simulink model "gravity"  (R2023a)
settings: Solver=FixedStepAuto  StartTime=0.0  StopTime=10.0  FixedStep=0.001  RelTol=1e-3
libraries: matrix_library x2
settings Model: Creator=romanos  LastModifiedBy=romanos
settings DataIOCC: ExternalInput="X_ecef,  R"  LoadExternalInput=on

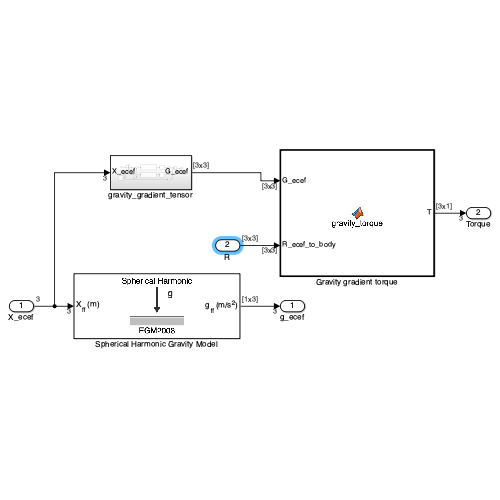
[thumbnail: Simulink's stored preview of the top-level diagram]
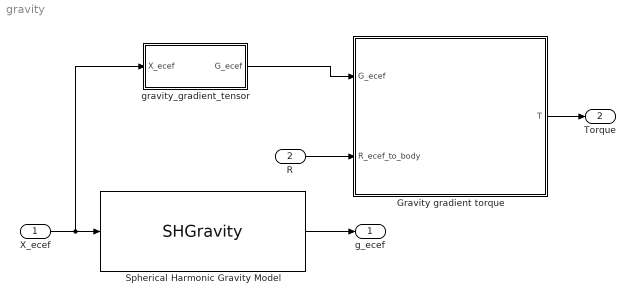
== system gravity ==
  X_ecef : Inport  PortDimensions=3
  R : Inport  Port=2  PortDimensions=[3 3]  Interpolate=off
  Gravity gradient torque : MATLAB Function  TreatAsAtomicUnit=on
  Spherical Harmonic Gravity Model : SHGravity
  gravity_gradient_tensor : Subsystem
  g_ecef : Outport  PortDimensions=3
  Torque : Outport  Port=2  PortDimensions=3
  wires:
  Gravity gradient torque/1(T) -> Torque/1
  X_ecef/1 -> Spherical Harmonic Gravity Model/1, gravity_gradient_tensor/1(X_ecef)
  Spherical Harmonic Gravity Model/1 -> g_ecef/1
  R/1 -> Gravity gradient torque/2(R_ecef_to_body)
  gravity_gradient_tensor/1(G_ecef) -> Gravity gradient torque/1(G_ecef)

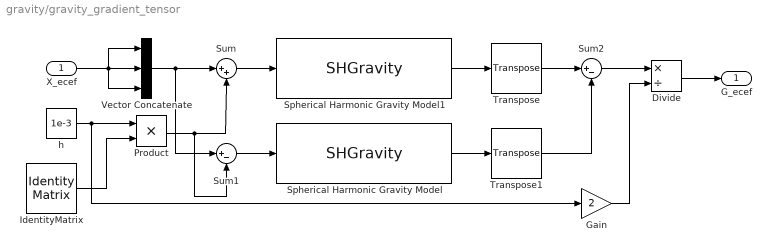
== system gravity/gravity_gradient_tensor ==
  X_ecef : Inport
  Divide : Product  Inputs=*/
  Gain : Gain  Gain=2
  IdentityMatrix : IdentityMatrix  OutputDimensions=3
  Product : Product
  Spherical Harmonic Gravity Model : SHGravity
  Spherical Harmonic Gravity Model1 : SHGravity
  Sum : Sum  Inputs=|++
  Sum1 : Sum  Inputs=|+-
  Sum2 : Sum  Inputs=|+-
  Transpose : matrix_library/Transpose
  Transpose1 : matrix_library/Transpose
  Vector Concatenate : Concatenate  NumInputs=3  Mode=Multidimensional array  ConcatenateDimension=2
  h : Constant  Value=1e-3
  G_ecef : Outport  PortDimensions=[3 3]
  wires:
  Divide/1 -> G_ecef/1
  Sum2/1 -> Divide/1
  Transpose/1 -> Sum2/1
  Gain/1 -> Divide/2
  Transpose1/1 -> Sum2/2
  Sum1/1 -> Spherical Harmonic Gravity Model/1
  Spherical Harmonic Gravity Model/1 -> Transpose1/1
  Sum/1 -> Spherical Harmonic Gravity Model1/1
  Product/1 -> Sum/2, Sum1/2
  h/1 -> Product/1, Gain/1
  Vector Concatenate/1 -> Sum1/1, Sum/1
  Spherical Harmonic Gravity Model1/1 -> Transpose/1
  IdentityMatrix/1 -> Product/2
  X_ecef/1 -> Vector Concatenate/1, Vector Concatenate/3, Vector Concatenate/2

== matlab function gravity/Gravity gradient torque ==
  data: G_ecef input; T output; R_ecef_to_body input; I parameter
function T   = gravity_torque(G_ecef, R_ecef_to_body, I) %#codegen
    G_body = R_ecef_to_body' * G_ecef * R_ecef_to_body;
    T = zeros(3,1);
    T(1) = G_body(2,3) * (I(3,3) - I(2,2)) + G_body(1,3) * I(1,2) - G_body(1,2) * I(1,3) + I(2,3) * (G_body(3,3) - G_body(2,2));
    T(2) = G_body(1,3) * (I(1,1) - I(3,3)) - G_body(2,3) * I(1,2) + G_body(1,2) * I(2,3) + I(1,3) * (G_body(1,1) - G_body(3,3));
    T(3) = G_body(1,2) * (I(2,2) - I(1,1)) + G_body(2,3) * I(1,3) - G_body(1,3) * I(2,3) + I(1,2) * (G_body(2,2) - G_body(1,1));
end
